simulink model "pendule_inv_capteur_etu"  (R2019a)
settings: Solver=VariableStepAuto  StartTime=0.0  StopTime=10.0  RelTol=1e-3
values from neighbouring files (symbols this model uses):
  g = 9.81    [simu_pendule_inv_capteur_etu.m]    (also in simu_pendule_inv_echant_etu.m; simu_pendule_inv_etu.m)
  K = [10 1]    [simu_pendule_inv_capteur_etu.m]    (also in simu_pendule_inv_echant_etu.m = [30 10]; simu_pendule_inv_etu.m = [30 10])
  l = 10    [simu_pendule_inv_capteur_etu.m]    (also in simu_pendule_inv_echant_etu.m; simu_pendule_inv_etu.m)
  ue = 0    [simu_pendule_inv_capteur_etu.m]    (also in simu_pendule_inv_echant_etu.m; simu_pendule_inv_etu.m)
  x0 = [pi/20 0]'    [simu_pendule_inv_capteur_etu.m]    (also in simu_pendule_inv_echant_etu.m; simu_pendule_inv_etu.m = [pi/10 0]')
  xe = [0 0]'    [simu_pendule_inv_capteur_etu.m]    (also in simu_pendule_inv_echant_etu.m; simu_pendule_inv_etu.m)
settings Model: Creator=aakby  LastModifiedBy=hmoudden

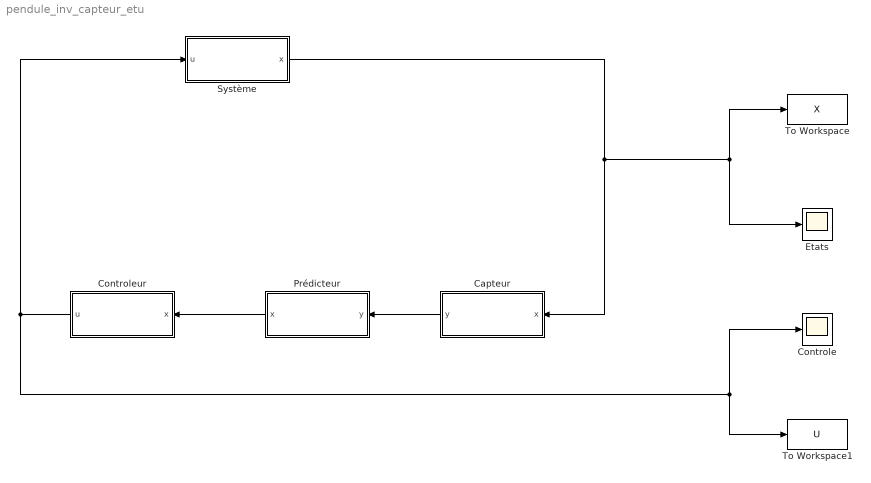
== system pendule_inv_capteur_etu ==
  Capteur : Subsystem
  Controle : Scope
  Controleur : Subsystem
  Etats : Scope
  Prédicteur : Subsystem
  Système : Subsystem
  To Workspace : ToWorkspace  VariableName=X  SaveFormat=Timeseries  SampleTime=-1
  To Workspace1 : ToWorkspace  VariableName=U  SaveFormat=Timeseries  SampleTime=-1
  wires:
  Système/1(x) -> Capteur/1(x), Etats/1, To Workspace/1
  Controleur/1(u) -> To Workspace1/1, Controle/1, Système/1(u)
  Prédicteur/1("x ") -> Controleur/1("x ")
  Capteur/1(y) -> Prédicteur/1("y ")

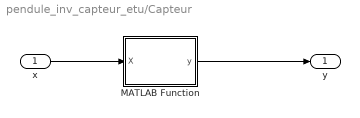
== system pendule_inv_capteur_etu/Capteur ==
  x : Inport
  MATLAB Function : MATLAB Function  TreatAsAtomicUnit=on
  y : Outport
  wires:
  x/1 -> MATLAB Function/1(X)
  MATLAB Function/1(y) -> y/1

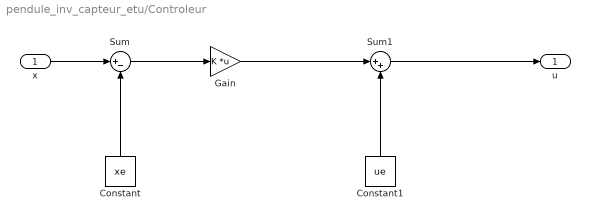
== system pendule_inv_capteur_etu/Controleur ==
  "x " : Inport
  Constant : Constant  Value=xe
  Constant1 : Constant  Value=ue
  Gain : Gain  Gain=K  Multiplication=Matrix(K*u)
  Sum : Sum  Inputs=|+-
  Sum1 : Sum  Inputs=|++
  u : Outport
  wires:
  "x "/1 -> Sum/1
  Constant/1 -> Sum/2
  Sum/1 -> Gain/1
  Gain/1 -> Sum1/1
  Constant1/1 -> Sum1/2
  Sum1/1 -> u/1

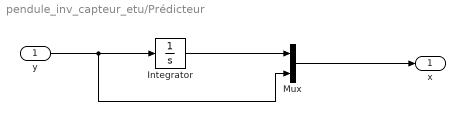
== system pendule_inv_capteur_etu/Prédicteur ==
  "y " : Inport
  Integrator : Integrator  InitialCondition=x0(1)
  Mux : Mux  Inputs=2
  "x " : Outport
  wires:
  Integrator/1 -> Mux/1
  "y "/1 -> Mux/2, Integrator/1
  Mux/1 -> "x "/1

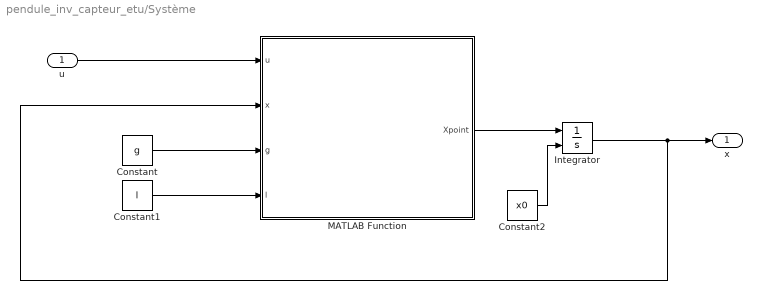
== system pendule_inv_capteur_etu/Système ==
  u : Inport
  Constant : Constant  Value=g
  Constant1 : Constant  Value=l
  Constant2 : Constant  Value=x0
  Integrator : Integrator  InitialConditionSource=external
  MATLAB Function : MATLAB Function  TreatAsAtomicUnit=on
  x : Outport
  wires:
  u/1 -> MATLAB Function/1(u)
  MATLAB Function/1(Xpoint) -> Integrator/1
  Integrator/1 -> x/1, MATLAB Function/2(x)
  Constant1/1 -> MATLAB Function/4(l)
  Constant/1 -> MATLAB Function/3(g)
  Constant2/1 -> Integrator/2

== matlab function pendule_inv_capteur_etu/Capteur/MATLAB Function ==
  data: X input; y output
function y = fcn(X)

y = X(2);

== matlab function pendule_inv_capteur_etu/Système/MATLAB Function ==
  data: u input; Xpoint output; x input; g input; l input
function Xpoint = fcn(u,x,g,l)

Xpoint = [x(2) g/l*sin(x(1))-cos(x(1))*u/l]';
